simulink model "closedloop_model_conditWindup"  (R2024a)
settings: Solver=VariableStepAuto  StartTime=0.0  StopTime=20  RelTol=1e-3
undefined symbols (not defined in the file): Kp, Td, Ti
libraries: cstblocks x2
settings Model: SimulationMode=accelerator  Creator=thoma  LastModifiedBy=thoma

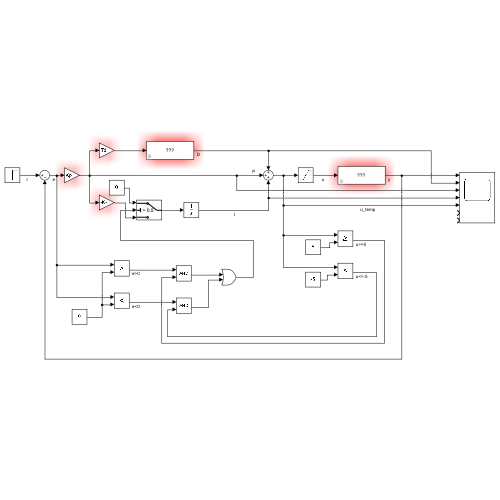
[thumbnail: Simulink's stored preview of the top-level diagram]
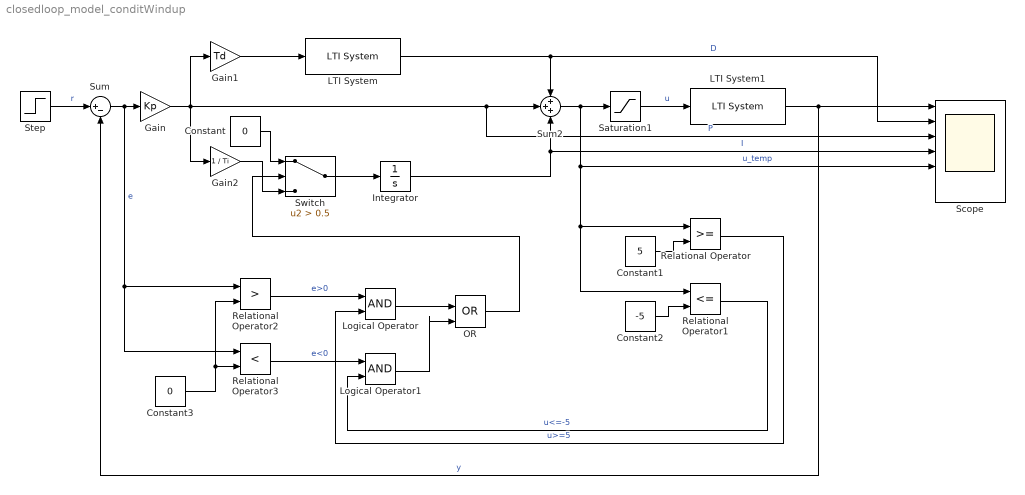
== system closedloop_model_conditWindup ==
  Constant : Constant  Value=0
  Constant1 : Constant  Value=5
  Constant2 : Constant  Value=-5
  Constant3 : Constant  Value=0
  Gain : Gain  Gain=Kp
  Gain1 : Gain  Gain=Td
  Gain2 : Gain  Gain=1 / Ti
  Integrator : Integrator
  LTI System : cstblocks/LTI System  sys=F  IC=[]  PadeOrder=0
  LTI System1 : cstblocks/LTI System  sys=G  IC=[]  PadeOrder=0
  Logical Operator : Logic  AllPortsSameDT=off  OutDataTypeStr=boolean
  Logical Operator1 : Logic  AllPortsSameDT=off  OutDataTypeStr=boolean
  OR : Logic  Operator=OR  IconShape=distinctive  AllPortsSameDT=off  OutDataTypeStr=boolean
  Relational Operator : RelationalOperator  OutDataTypeStr=boolean  RndMeth=Simplest  InputSameDT=off
  Relational Operator1 : RelationalOperator  Operator=<=  OutDataTypeStr=boolean  RndMeth=Simplest  InputSameDT=off
  Relational Operator2 : RelationalOperator  Operator=>  OutDataTypeStr=boolean  RndMeth=Simplest  InputSameDT=off
  Relational Operator3 : RelationalOperator  Operator=<  OutDataTypeStr=boolean  RndMeth=Simplest  InputSameDT=off
  Saturation1 : Saturate  UpperLimit=5  LowerLimit=-5
  Scope : Scope  NumInputPorts=7
  Step : Step  Time=0  SampleTime=0
  Sum : Sum  Inputs=|+-
  Sum2 : Sum  Inputs=+++
  Switch : Switch  Criteria=u2 > Threshold  Threshold=0.5  SaturateOnIntegerOverflow=off  InputSameDT=off
  wires:
  Gain/1 -> Scope/3, Sum2/2, Gain1/1, Gain2/1  "P"
  Step/1 -> Sum/1  "r"
  Gain1/1 -> LTI System/1
  LTI System/1 -> Sum2/1, Scope/2  "D"
  LTI System1/1 -> Sum/2, Scope/1  "y"
  Sum2/1 -> Relational Operator1/1, Relational Operator/1, Scope/5, Saturation1/1  "u_temp"
  Saturation1/1 -> LTI System1/1  "u"
  Integrator/1 -> Scope/4, Sum2/3  "I"
  Sum/1 -> Relational Operator2/1, Relational Operator3/1, Gain/1  "e"
  Switch/1 -> Integrator/1
  Gain2/1 -> Switch/3
  Constant1/1 -> Relational Operator/2
  Constant2/1 -> Relational Operator1/2
  Constant3/1 -> Relational Operator2/2, Relational Operator3/2
  Relational Operator/1 -> Logical Operator/2  "u>=5"
  Relational Operator1/1 -> Logical Operator1/2  "u<=-5"
  Relational Operator3/1 -> Logical Operator1/1  "e<0"
  Logical Operator/1 -> OR/1
  Logical Operator1/1 -> OR/2
  OR/1 -> Switch/2
  Relational Operator2/1 -> Logical Operator/1  "e>0"
  Constant/1 -> Switch/1
